simulink model "secondcontroller"  (R2021b)
settings: Solver=VariableStepAuto  StartTime=0.0  StopTime=10.0  RelTol=1e-3
libraries: dspsrcs4 x1
settings Model: Creator=Asus  LastModifiedBy=Matina Kaviani
settings SolverCC: AlgebraicLoopSolver=TrustRegion
settings DebuggingCC: SFMachineParentedDataDiag=warning

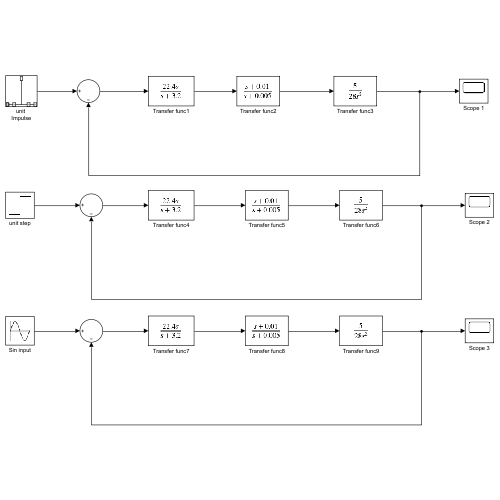
[thumbnail: Simulink's stored preview of the top-level diagram]
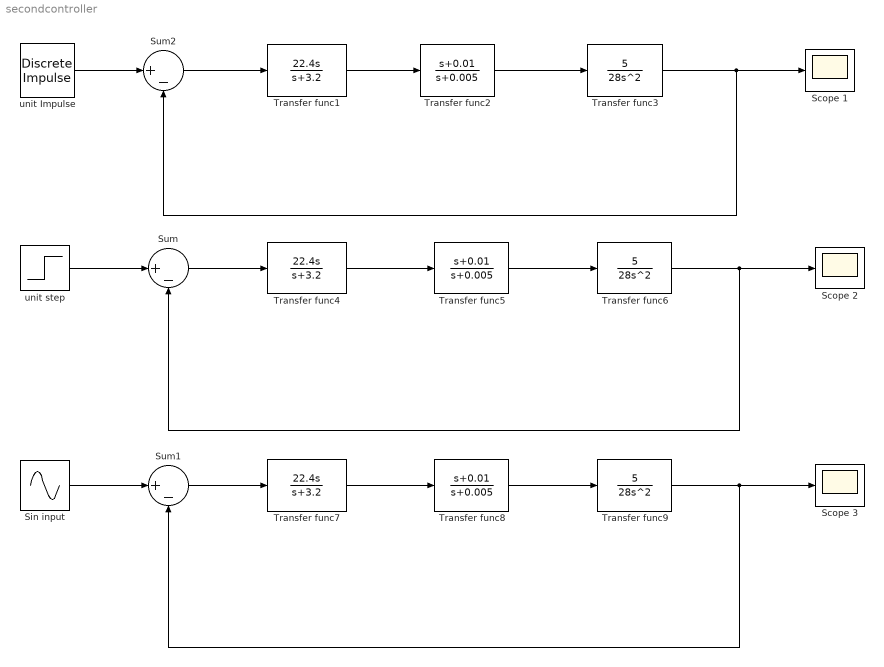
== system secondcontroller ==
  Scope 1 : Scope
  Scope 2 : Scope
  Scope 3 : Scope
  Sin input : Sin  Frequency=2*pi  SampleTime=0
  Sum : Sum  Inputs=|+-
  Sum1 : Sum  Inputs=|+-
  Sum2 : Sum  Inputs=|+-
  Transfer func1 : TransferFcn  Numerator=[22.4 0]  Denominator=[1 3.2]
  Transfer func2 : TransferFcn  Numerator=[1 0.01]  Denominator=[1 0.005]
  Transfer func3 : TransferFcn  Numerator=[0 5]  Denominator=[28 0 0]
  Transfer func4 : TransferFcn  Numerator=[22.4 0]  Denominator=[1 3.2]
  Transfer func5 : TransferFcn  Numerator=[1 0.01]  Denominator=[1 0.005]
  Transfer func6 : TransferFcn  Numerator=[0 5]  Denominator=[28 0 0]
  Transfer func7 : TransferFcn  Numerator=[22.4 0]  Denominator=[1 3.2]
  Transfer func8 : TransferFcn  Numerator=[1 0.01]  Denominator=[1 0.005]
  Transfer func9 : TransferFcn  Numerator=[0 5]  Denominator=[28 0 0]
  unit Impulse : dspsrcs4/Discrete  Impulse  Delay=0  SampleTime=1  FrameSample=1  OutputFrames=off  dataType=double  isSigned=on  wordLen=16  udDataType=sfix(16)  fracBitsMode=Best precision  numFracBits=15  OutDataTypeStr=double  LastOutDataTypeStr=double
  unit step : Step  After=2  SampleTime=0
  wires:
  unit step/1 -> Sum/1
  Sum/1 -> Transfer func4/1
  Transfer func4/1 -> Transfer func5/1
  Transfer func5/1 -> Transfer func6/1
  Transfer func6/1 -> Sum/2, Scope 2/1
  Sum1/1 -> Transfer func7/1
  Transfer func7/1 -> Transfer func8/1
  Transfer func9/1 -> Sum1/2, Scope 3/1
  Transfer func8/1 -> Transfer func9/1
  Sin input/1 -> Sum1/1
  unit Impulse/1 -> Sum2/1
  Sum2/1 -> Transfer func1/1
  Transfer func1/1 -> Transfer func2/1
  Transfer func2/1 -> Transfer func3/1
  Transfer func3/1 -> Sum2/2, Scope 1/1
